simulink model "final_model"  (R2023b)
settings: Solver=VariableStepAuto  StartTime=0.0  StopTime=200  RelTol=1e-3
(part 2 of 3)

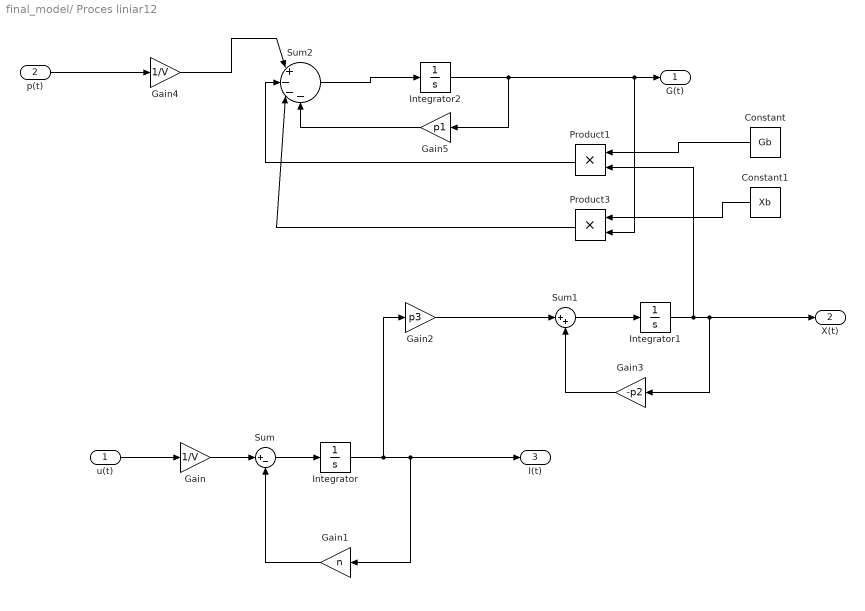
== system final_model/ Proces liniar12 ==
  " u(t)" : Inport
  p(t) : Inport  Port=2
  Constant : Constant  Value=Gb
  Constant1 : Constant  Value=Xb
  Gain : Gain  Gain=1/V
  Gain1 : Gain  Gain=n
  Gain2 : Gain  Gain=p3
  Gain3 : Gain  Gain=-p2
  Gain4 : Gain  Gain=1/V
  Gain5 : Gain  Gain=p1
  Integrator : Integrator
  Integrator1 : Integrator
  Integrator2 : Integrator  InitialCondition=G0
  Product1 : Product
  Product3 : Product
  Sum : Sum  Inputs=|+-
  Sum1 : Sum  Inputs=|++
  Sum2 : Sum  Inputs=|+---
  " G(t)" : Outport
  X(t) : Outport  Port=2
  I(t) : Outport  Port=3
  wires:
  Gain2/1 -> Sum1/1
  Gain/1 -> Sum/1
  " u(t)"/1 -> Gain/1
  Sum/1 -> Integrator/1
  Gain1/1 -> Sum/2
  Integrator2/1 -> Product3/2, " G(t)"/1, Gain5/1
  Integrator1/1 -> Product1/2, Gain3/1, X(t)/1
  Integrator/1 -> Gain2/1, I(t)/1, Gain1/1
  Gain3/1 -> Sum1/2
  Gain4/1 -> Sum2/1
  Gain5/1 -> Sum2/4
  p(t)/1 -> Gain4/1
  Sum1/1 -> Integrator1/1
  Sum2/1 -> Integrator2/1
  Constant/1 -> Product1/1
  Constant1/1 -> Product3/1
  Product3/1 -> Sum2/3
  Product1/1 -> Sum2/2

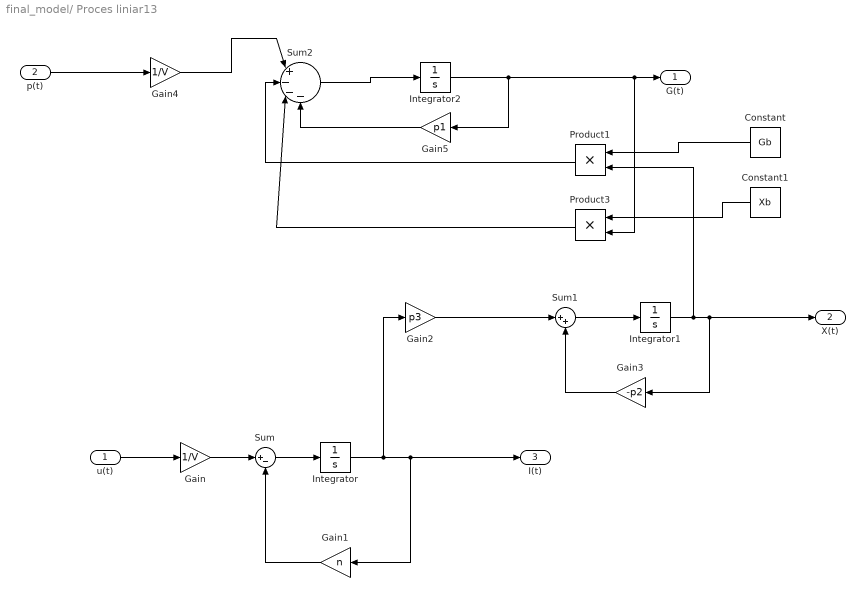
== system final_model/ Proces liniar13 ==
  " u(t)" : Inport
  p(t) : Inport  Port=2
  Constant : Constant  Value=Gb
  Constant1 : Constant  Value=Xb
  Gain : Gain  Gain=1/V
  Gain1 : Gain  Gain=n
  Gain2 : Gain  Gain=p3
  Gain3 : Gain  Gain=-p2
  Gain4 : Gain  Gain=1/V
  Gain5 : Gain  Gain=p1
  Integrator : Integrator
  Integrator1 : Integrator
  Integrator2 : Integrator  InitialCondition=G0
  Product1 : Product
  Product3 : Product
  Sum : Sum  Inputs=|+-
  Sum1 : Sum  Inputs=|++
  Sum2 : Sum  Inputs=|+---
  " G(t)" : Outport
  X(t) : Outport  Port=2
  I(t) : Outport  Port=3
  wires:
  Gain2/1 -> Sum1/1
  Gain/1 -> Sum/1
  " u(t)"/1 -> Gain/1
  Sum/1 -> Integrator/1
  Gain1/1 -> Sum/2
  Integrator2/1 -> Product3/2, " G(t)"/1, Gain5/1
  Integrator1/1 -> Product1/2, Gain3/1, X(t)/1
  Integrator/1 -> Gain2/1, I(t)/1, Gain1/1
  Gain3/1 -> Sum1/2
  Gain4/1 -> Sum2/1
  Gain5/1 -> Sum2/4
  p(t)/1 -> Gain4/1
  Sum1/1 -> Integrator1/1
  Sum2/1 -> Integrator2/1
  Constant/1 -> Product1/1
  Constant1/1 -> Product3/1
  Product3/1 -> Sum2/3
  Product1/1 -> Sum2/2

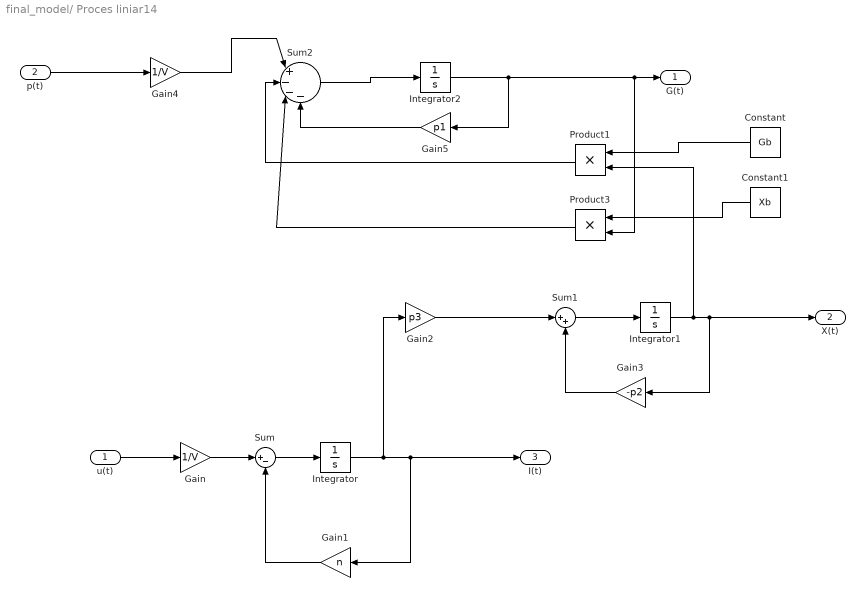
== system final_model/ Proces liniar14 ==
  " u(t)" : Inport
  p(t) : Inport  Port=2
  Constant : Constant  Value=Gb
  Constant1 : Constant  Value=Xb
  Gain : Gain  Gain=1/V
  Gain1 : Gain  Gain=n
  Gain2 : Gain  Gain=p3
  Gain3 : Gain  Gain=-p2
  Gain4 : Gain  Gain=1/V
  Gain5 : Gain  Gain=p1
  Integrator : Integrator
  Integrator1 : Integrator
  Integrator2 : Integrator  InitialCondition=G0
  Product1 : Product
  Product3 : Product
  Sum : Sum  Inputs=|+-
  Sum1 : Sum  Inputs=|++
  Sum2 : Sum  Inputs=|+---
  " G(t)" : Outport
  X(t) : Outport  Port=2
  I(t) : Outport  Port=3
  wires:
  Gain2/1 -> Sum1/1
  Gain/1 -> Sum/1
  " u(t)"/1 -> Gain/1
  Sum/1 -> Integrator/1
  Gain1/1 -> Sum/2
  Integrator2/1 -> Product3/2, " G(t)"/1, Gain5/1
  Integrator1/1 -> Product1/2, Gain3/1, X(t)/1
  Integrator/1 -> Gain2/1, I(t)/1, Gain1/1
  Gain3/1 -> Sum1/2
  Gain4/1 -> Sum2/1
  Gain5/1 -> Sum2/4
  p(t)/1 -> Gain4/1
  Sum1/1 -> Integrator1/1
  Sum2/1 -> Integrator2/1
  Constant/1 -> Product1/1
  Constant1/1 -> Product3/1
  Product3/1 -> Sum2/3
  Product1/1 -> Sum2/2

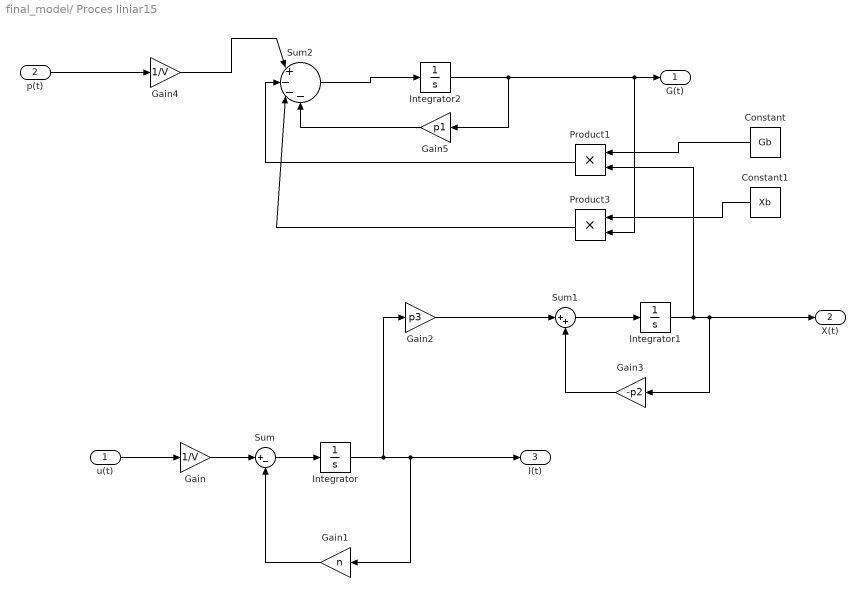
== system final_model/ Proces liniar15 ==
  " u(t)" : Inport
  p(t) : Inport  Port=2
  Constant : Constant  Value=Gb
  Constant1 : Constant  Value=Xb
  Gain : Gain  Gain=1/V
  Gain1 : Gain  Gain=n
  Gain2 : Gain  Gain=p3
  Gain3 : Gain  Gain=-p2
  Gain4 : Gain  Gain=1/V
  Gain5 : Gain  Gain=p1
  Integrator : Integrator
  Integrator1 : Integrator
  Integrator2 : Integrator  InitialCondition=G0
  Product1 : Product
  Product3 : Product
  Sum : Sum  Inputs=|+-
  Sum1 : Sum  Inputs=|++
  Sum2 : Sum  Inputs=|+---
  " G(t)" : Outport
  X(t) : Outport  Port=2
  I(t) : Outport  Port=3
  wires:
  Gain2/1 -> Sum1/1
  Gain/1 -> Sum/1
  " u(t)"/1 -> Gain/1
  Sum/1 -> Integrator/1
  Gain1/1 -> Sum/2
  Integrator2/1 -> Product3/2, " G(t)"/1, Gain5/1
  Integrator1/1 -> Product1/2, Gain3/1, X(t)/1
  Integrator/1 -> Gain2/1, I(t)/1, Gain1/1
  Gain3/1 -> Sum1/2
  Gain4/1 -> Sum2/1
  Gain5/1 -> Sum2/4
  p(t)/1 -> Gain4/1
  Sum1/1 -> Integrator1/1
  Sum2/1 -> Integrator2/1
  Constant/1 -> Product1/1
  Constant1/1 -> Product3/1
  Product3/1 -> Sum2/3
  Product1/1 -> Sum2/2

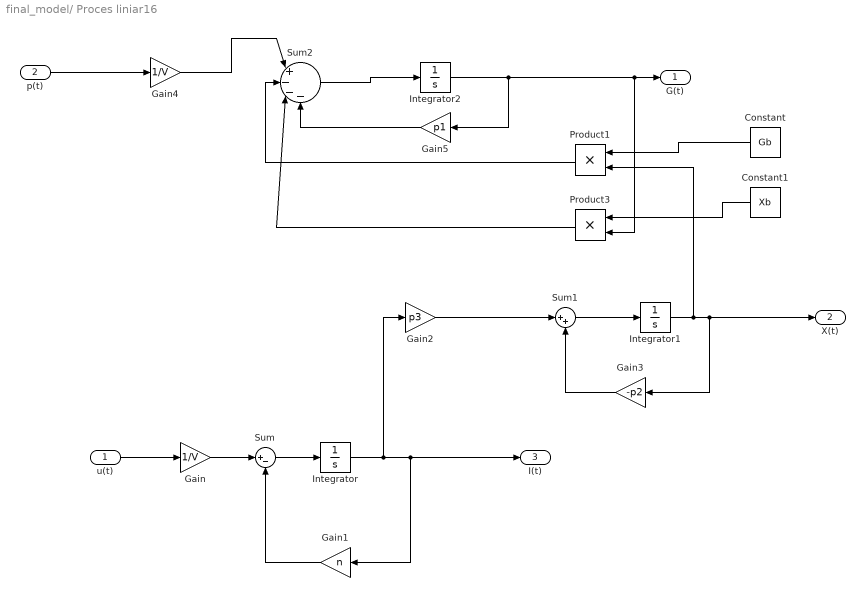
== system final_model/ Proces liniar16 ==
  " u(t)" : Inport
  p(t) : Inport  Port=2
  Constant : Constant  Value=Gb
  Constant1 : Constant  Value=Xb
  Gain : Gain  Gain=1/V
  Gain1 : Gain  Gain=n
  Gain2 : Gain  Gain=p3
  Gain3 : Gain  Gain=-p2
  Gain4 : Gain  Gain=1/V
  Gain5 : Gain  Gain=p1
  Integrator : Integrator
  Integrator1 : Integrator
  Integrator2 : Integrator  InitialCondition=G0
  Product1 : Product
  Product3 : Product
  Sum : Sum  Inputs=|+-
  Sum1 : Sum  Inputs=|++
  Sum2 : Sum  Inputs=|+---
  " G(t)" : Outport
  X(t) : Outport  Port=2
  I(t) : Outport  Port=3
  wires:
  Gain2/1 -> Sum1/1
  Gain/1 -> Sum/1
  " u(t)"/1 -> Gain/1
  Sum/1 -> Integrator/1
  Gain1/1 -> Sum/2
  Integrator2/1 -> Product3/2, " G(t)"/1, Gain5/1
  Integrator1/1 -> Product1/2, Gain3/1, X(t)/1
  Integrator/1 -> Gain2/1, I(t)/1, Gain1/1
  Gain3/1 -> Sum1/2
  Gain4/1 -> Sum2/1
  Gain5/1 -> Sum2/4
  p(t)/1 -> Gain4/1
  Sum1/1 -> Integrator1/1
  Sum2/1 -> Integrator2/1
  Constant/1 -> Product1/1
  Constant1/1 -> Product3/1
  Product3/1 -> Sum2/3
  Product1/1 -> Sum2/2

== system final_model/ Proces liniar17 ==
  " u(t)" : Inport
  p(t) : Inport  Port=2
  Constant : Constant  Value=Gb
  Constant1 : Constant  Value=Xb
  Gain : Gain  Gain=1/V
  Gain1 : Gain  Gain=n
  Gain2 : Gain  Gain=p3
  Gain3 : Gain  Gain=-p2
  Gain4 : Gain  Gain=1/V
  Gain5 : Gain  Gain=p1
  Integrator : Integrator
  Integrator1 : Integrator
  Integrator2 : Integrator  InitialCondition=G0
  Product1 : Product
  Product3 : Product
  Sum : Sum  Inputs=|+-
  Sum1 : Sum  Inputs=|++
  Sum2 : Sum  Inputs=|+---
  " G(t)" : Outport
  X(t) : Outport  Port=2
  I(t) : Outport  Port=3
  wires:
  Gain2/1 -> Sum1/1
  Gain/1 -> Sum/1
  " u(t)"/1 -> Gain/1
  Sum/1 -> Integrator/1
  Gain1/1 -> Sum/2
  Integrator2/1 -> Product3/2, " G(t)"/1, Gain5/1
  Integrator1/1 -> Product1/2, Gain3/1, X(t)/1
  Integrator/1 -> Gain2/1, I(t)/1, Gain1/1
  Gain3/1 -> Sum1/2
  Gain4/1 -> Sum2/1
  Gain5/1 -> Sum2/4
  p(t)/1 -> Gain4/1
  Sum1/1 -> Integrator1/1
  Sum2/1 -> Integrator2/1
  Constant/1 -> Product1/1
  Constant1/1 -> Product3/1
  Product3/1 -> Sum2/3
  Product1/1 -> Sum2/2

== system final_model/ Proces liniar18 ==
  " u(t)" : Inport
  p(t) : Inport  Port=2
  Constant : Constant  Value=Gb
  Constant1 : Constant  Value=Xb
  Gain : Gain  Gain=1/V
  Gain1 : Gain  Gain=n
  Gain2 : Gain  Gain=p3
  Gain3 : Gain  Gain=-p2
  Gain4 : Gain  Gain=1/V
  Gain5 : Gain  Gain=p1
  Integrator : Integrator
  Integrator1 : Integrator
  Integrator2 : Integrator  InitialCondition=G0
  Product1 : Product
  Product3 : Product
  Sum : Sum  Inputs=|+-
  Sum1 : Sum  Inputs=|++
  Sum2 : Sum  Inputs=|+---
  " G(t)" : Outport
  X(t) : Outport  Port=2
  I(t) : Outport  Port=3
  wires:
  Gain2/1 -> Sum1/1
  Gain/1 -> Sum/1
  " u(t)"/1 -> Gain/1
  Sum/1 -> Integrator/1
  Gain1/1 -> Sum/2
  Integrator2/1 -> Product3/2, " G(t)"/1, Gain5/1
  Integrator1/1 -> Product1/2, Gain3/1, X(t)/1
  Integrator/1 -> Gain2/1, I(t)/1, Gain1/1
  Gain3/1 -> Sum1/2
  Gain4/1 -> Sum2/1
  Gain5/1 -> Sum2/4
  p(t)/1 -> Gain4/1
  Sum1/1 -> Integrator1/1
  Sum2/1 -> Integrator2/1
  Constant/1 -> Product1/1
  Constant1/1 -> Product3/1
  Product3/1 -> Sum2/3
  Product1/1 -> Sum2/2

== system final_model/ Proces liniar19 ==
  " u(t)" : Inport
  p(t) : Inport  Port=2
  Constant : Constant  Value=Gb
  Constant1 : Constant  Value=Xb
  Gain : Gain  Gain=1/V
  Gain1 : Gain  Gain=n
  Gain2 : Gain  Gain=p3
  Gain3 : Gain  Gain=-p2
  Gain4 : Gain  Gain=1/V
  Gain5 : Gain  Gain=p1
  Integrator : Integrator
  Integrator1 : Integrator
  Integrator2 : Integrator  InitialCondition=G0
  Product1 : Product
  Product3 : Product
  Sum : Sum  Inputs=|+-
  Sum1 : Sum  Inputs=|++
  Sum2 : Sum  Inputs=|+---
  " G(t)" : Outport
  X(t) : Outport  Port=2
  I(t) : Outport  Port=3
  wires:
  Gain2/1 -> Sum1/1
  Gain/1 -> Sum/1
  " u(t)"/1 -> Gain/1
  Sum/1 -> Integrator/1
  Gain1/1 -> Sum/2
  Integrator2/1 -> Product3/2, " G(t)"/1, Gain5/1
  Integrator1/1 -> Product1/2, Gain3/1, X(t)/1
  Integrator/1 -> Gain2/1, I(t)/1, Gain1/1
  Gain3/1 -> Sum1/2
  Gain4/1 -> Sum2/1
  Gain5/1 -> Sum2/4
  p(t)/1 -> Gain4/1
  Sum1/1 -> Integrator1/1
  Sum2/1 -> Integrator2/1
  Constant/1 -> Product1/1
  Constant1/1 -> Product3/1
  Product3/1 -> Sum2/3
  Product1/1 -> Sum2/2

== system final_model/ Proces liniar2 ==
  " u(t)" : Inport
  p(t) : Inport  Port=2
  Constant : Constant  Value=Gb
  Constant1 : Constant  Value=Xb
  Gain : Gain  Gain=1/V
  Gain1 : Gain  Gain=n
  Gain2 : Gain  Gain=p3
  Gain3 : Gain  Gain=-p2
  Gain4 : Gain  Gain=1/V
  Gain5 : Gain  Gain=p1
  Integrator : Integrator
  Integrator1 : Integrator
  Integrator2 : Integrator  InitialCondition=G0
  Product1 : Product
  Product3 : Product
  Sum : Sum  Inputs=|+-
  Sum1 : Sum  Inputs=|++
  Sum2 : Sum  Inputs=|+---
  " G(t)" : Outport
  X(t) : Outport  Port=2
  I(t) : Outport  Port=3
  wires:
  Gain2/1 -> Sum1/1
  Gain/1 -> Sum/1
  " u(t)"/1 -> Gain/1
  Sum/1 -> Integrator/1
  Gain1/1 -> Sum/2
  Integrator2/1 -> Product3/2, " G(t)"/1, Gain5/1
  Integrator1/1 -> Product1/2, Gain3/1, X(t)/1
  Integrator/1 -> Gain2/1, I(t)/1, Gain1/1
  Gain3/1 -> Sum1/2
  Gain4/1 -> Sum2/1
  Gain5/1 -> Sum2/4
  p(t)/1 -> Gain4/1
  Sum1/1 -> Integrator1/1
  Sum2/1 -> Integrator2/1
  Constant/1 -> Product1/1
  Constant1/1 -> Product3/1
  Product3/1 -> Sum2/3
  Product1/1 -> Sum2/2

== system final_model/ Proces liniar20 ==
  " u(t)" : Inport
  p(t) : Inport  Port=2
  Constant : Constant  Value=Gb
  Constant1 : Constant  Value=Xb
  Gain : Gain  Gain=1/V
  Gain1 : Gain  Gain=n
  Gain2 : Gain  Gain=p3
  Gain3 : Gain  Gain=-p2
  Gain4 : Gain  Gain=1/V
  Gain5 : Gain  Gain=p1
  Integrator : Integrator
  Integrator1 : Integrator
  Integrator2 : Integrator  InitialCondition=G0
  Product1 : Product
  Product3 : Product
  Sum : Sum  Inputs=|+-
  Sum1 : Sum  Inputs=|++
  Sum2 : Sum  Inputs=|+---
  " G(t)" : Outport
  X(t) : Outport  Port=2
  I(t) : Outport  Port=3
  wires:
  Gain2/1 -> Sum1/1
  Gain/1 -> Sum/1
  " u(t)"/1 -> Gain/1
  Sum/1 -> Integrator/1
  Gain1/1 -> Sum/2
  Integrator2/1 -> Product3/2, " G(t)"/1, Gain5/1
  Integrator1/1 -> Product1/2, Gain3/1, X(t)/1
  Integrator/1 -> Gain2/1, I(t)/1, Gain1/1
  Gain3/1 -> Sum1/2
  Gain4/1 -> Sum2/1
  Gain5/1 -> Sum2/4
  p(t)/1 -> Gain4/1
  Sum1/1 -> Integrator1/1
  Sum2/1 -> Integrator2/1
  Constant/1 -> Product1/1
  Constant1/1 -> Product3/1
  Product3/1 -> Sum2/3
  Product1/1 -> Sum2/2

== system final_model/ Proces liniar21 ==
  " u(t)" : Inport
  p(t) : Inport  Port=2
  Constant : Constant  Value=Gb
  Constant1 : Constant  Value=Xb
  Gain : Gain  Gain=1/V
  Gain1 : Gain  Gain=n
  Gain2 : Gain  Gain=p3
  Gain3 : Gain  Gain=-p2
  Gain4 : Gain  Gain=1/V
  Gain5 : Gain  Gain=p1
  Integrator : Integrator
  Integrator1 : Integrator
  Integrator2 : Integrator  InitialCondition=G0
  Product1 : Product
  Product3 : Product
  Sum : Sum  Inputs=|+-
  Sum1 : Sum  Inputs=|++
  Sum2 : Sum  Inputs=|+---
  " G(t)" : Outport
  X(t) : Outport  Port=2
  I(t) : Outport  Port=3
  wires:
  Gain2/1 -> Sum1/1
  Gain/1 -> Sum/1
  " u(t)"/1 -> Gain/1
  Sum/1 -> Integrator/1
  Gain1/1 -> Sum/2
  Integrator2/1 -> Product3/2, " G(t)"/1, Gain5/1
  Integrator1/1 -> Product1/2, Gain3/1, X(t)/1
  Integrator/1 -> Gain2/1, I(t)/1, Gain1/1
  Gain3/1 -> Sum1/2
  Gain4/1 -> Sum2/1
  Gain5/1 -> Sum2/4
  p(t)/1 -> Gain4/1
  Sum1/1 -> Integrator1/1
  Sum2/1 -> Integrator2/1
  Constant/1 -> Product1/1
  Constant1/1 -> Product3/1
  Product3/1 -> Sum2/3
  Product1/1 -> Sum2/2

== system final_model/ Proces liniar22 ==
  " u(t)" : Inport
  p(t) : Inport  Port=2
  Constant : Constant  Value=Gb
  Constant1 : Constant  Value=Xb
  Gain : Gain  Gain=1/V
  Gain1 : Gain  Gain=n
  Gain2 : Gain  Gain=p3
  Gain3 : Gain  Gain=-p2
  Gain4 : Gain  Gain=1/V
  Gain5 : Gain  Gain=p1
  Integrator : Integrator
  Integrator1 : Integrator
  Integrator2 : Integrator  InitialCondition=G0
  Product1 : Product
  Product3 : Product
  Sum : Sum  Inputs=|+-
  Sum1 : Sum  Inputs=|++
  Sum2 : Sum  Inputs=|+---
  " G(t)" : Outport
  X(t) : Outport  Port=2
  I(t) : Outport  Port=3
  wires:
  Gain2/1 -> Sum1/1
  Gain/1 -> Sum/1
  " u(t)"/1 -> Gain/1
  Sum/1 -> Integrator/1
  Gain1/1 -> Sum/2
  Integrator2/1 -> Product3/2, " G(t)"/1, Gain5/1
  Integrator1/1 -> Product1/2, Gain3/1, X(t)/1
  Integrator/1 -> Gain2/1, I(t)/1, Gain1/1
  Gain3/1 -> Sum1/2
  Gain4/1 -> Sum2/1
  Gain5/1 -> Sum2/4
  p(t)/1 -> Gain4/1
  Sum1/1 -> Integrator1/1
  Sum2/1 -> Integrator2/1
  Constant/1 -> Product1/1
  Constant1/1 -> Product3/1
  Product3/1 -> Sum2/3
  Product1/1 -> Sum2/2

== system final_model/ Proces liniar23 ==
  " u(t)" : Inport
  p(t) : Inport  Port=2
  Constant : Constant  Value=Gb
  Constant1 : Constant  Value=Xb
  Gain : Gain  Gain=1/V
  Gain1 : Gain  Gain=n
  Gain2 : Gain  Gain=p3
  Gain3 : Gain  Gain=-p2
  Gain4 : Gain  Gain=1/V
  Gain5 : Gain  Gain=p1
  Integrator : Integrator
  Integrator1 : Integrator
  Integrator2 : Integrator  InitialCondition=G0
  Product1 : Product
  Product3 : Product
  Sum : Sum  Inputs=|+-
  Sum1 : Sum  Inputs=|++
  Sum2 : Sum  Inputs=|+---
  " G(t)" : Outport
  X(t) : Outport  Port=2
  I(t) : Outport  Port=3
  wires:
  Gain2/1 -> Sum1/1
  Gain/1 -> Sum/1
  " u(t)"/1 -> Gain/1
  Sum/1 -> Integrator/1
  Gain1/1 -> Sum/2
  Integrator2/1 -> Product3/2, " G(t)"/1, Gain5/1
  Integrator1/1 -> Product1/2, Gain3/1, X(t)/1
  Integrator/1 -> Gain2/1, I(t)/1, Gain1/1
  Gain3/1 -> Sum1/2
  Gain4/1 -> Sum2/1
  Gain5/1 -> Sum2/4
  p(t)/1 -> Gain4/1
  Sum1/1 -> Integrator1/1
  Sum2/1 -> Integrator2/1
  Constant/1 -> Product1/1
  Constant1/1 -> Product3/1
  Product3/1 -> Sum2/3
  Product1/1 -> Sum2/2

== system final_model/ Proces liniar24 ==
  " u(t)" : Inport
  p(t) : Inport  Port=2
  Constant : Constant  Value=Gb
  Constant1 : Constant  Value=Xb
  Gain : Gain  Gain=1/V
  Gain1 : Gain  Gain=n
  Gain2 : Gain  Gain=p3
  Gain3 : Gain  Gain=-p2
  Gain4 : Gain  Gain=1/V
  Gain5 : Gain  Gain=p1
  Integrator : Integrator
  Integrator1 : Integrator
  Integrator2 : Integrator  InitialCondition=G0
  Product1 : Product
  Product3 : Product
  Sum : Sum  Inputs=|+-
  Sum1 : Sum  Inputs=|++
  Sum2 : Sum  Inputs=|+---
  " G(t)" : Outport
  X(t) : Outport  Port=2
  I(t) : Outport  Port=3
  wires:
  Gain2/1 -> Sum1/1
  Gain/1 -> Sum/1
  " u(t)"/1 -> Gain/1
  Sum/1 -> Integrator/1
  Gain1/1 -> Sum/2
  Integrator2/1 -> Product3/2, " G(t)"/1, Gain5/1
  Integrator1/1 -> Product1/2, Gain3/1, X(t)/1
  Integrator/1 -> Gain2/1, I(t)/1, Gain1/1
  Gain3/1 -> Sum1/2
  Gain4/1 -> Sum2/1
  Gain5/1 -> Sum2/4
  p(t)/1 -> Gain4/1
  Sum1/1 -> Integrator1/1
  Sum2/1 -> Integrator2/1
  Constant/1 -> Product1/1
  Constant1/1 -> Product3/1
  Product3/1 -> Sum2/3
  Product1/1 -> Sum2/2

== system final_model/ Proces liniar25 ==
  " u(t)" : Inport
  p(t) : Inport  Port=2
  Constant : Constant  Value=Gb
  Constant1 : Constant  Value=Xb
  Gain : Gain  Gain=1/V
  Gain1 : Gain  Gain=n
  Gain2 : Gain  Gain=p3
  Gain3 : Gain  Gain=-p2
  Gain4 : Gain  Gain=1/V
  Gain5 : Gain  Gain=p1
  Integrator : Integrator
  Integrator1 : Integrator
  Integrator2 : Integrator  InitialCondition=G0
  Product1 : Product
  Product3 : Product
  Sum : Sum  Inputs=|+-
  Sum1 : Sum  Inputs=|++
  Sum2 : Sum  Inputs=|+---
  " G(t)" : Outport
  X(t) : Outport  Port=2
  I(t) : Outport  Port=3
  wires:
  Gain2/1 -> Sum1/1
  Gain/1 -> Sum/1
  " u(t)"/1 -> Gain/1
  Sum/1 -> Integrator/1
  Gain1/1 -> Sum/2
  Integrator2/1 -> Product3/2, " G(t)"/1, Gain5/1
  Integrator1/1 -> Product1/2, Gain3/1, X(t)/1
  Integrator/1 -> Gain2/1, I(t)/1, Gain1/1
  Gain3/1 -> Sum1/2
  Gain4/1 -> Sum2/1
  Gain5/1 -> Sum2/4
  p(t)/1 -> Gain4/1
  Sum1/1 -> Integrator1/1
  Sum2/1 -> Integrator2/1
  Constant/1 -> Product1/1
  Constant1/1 -> Product3/1
  Product3/1 -> Sum2/3
  Product1/1 -> Sum2/2

== system final_model/ Proces liniar26 ==
  " u(t)" : Inport
  p(t) : Inport  Port=2
  Constant : Constant  Value=Gb
  Constant1 : Constant  Value=Xb
  Gain : Gain  Gain=1/V
  Gain1 : Gain  Gain=n
  Gain2 : Gain  Gain=p3
  Gain3 : Gain  Gain=-p2
  Gain4 : Gain  Gain=1/V
  Gain5 : Gain  Gain=p1
  Integrator : Integrator
  Integrator1 : Integrator
  Integrator2 : Integrator  InitialCondition=G0
  Product1 : Product
  Product3 : Product
  Sum : Sum  Inputs=|+-
  Sum1 : Sum  Inputs=|++
  Sum2 : Sum  Inputs=|+---
  " G(t)" : Outport
  X(t) : Outport  Port=2
  I(t) : Outport  Port=3
  wires:
  Gain2/1 -> Sum1/1
  Gain/1 -> Sum/1
  " u(t)"/1 -> Gain/1
  Sum/1 -> Integrator/1
  Gain1/1 -> Sum/2
  Integrator2/1 -> Product3/2, " G(t)"/1, Gain5/1
  Integrator1/1 -> Product1/2, Gain3/1, X(t)/1
  Integrator/1 -> Gain2/1, I(t)/1, Gain1/1
  Gain3/1 -> Sum1/2
  Gain4/1 -> Sum2/1
  Gain5/1 -> Sum2/4
  p(t)/1 -> Gain4/1
  Sum1/1 -> Integrator1/1
  Sum2/1 -> Integrator2/1
  Constant/1 -> Product1/1
  Constant1/1 -> Product3/1
  Product3/1 -> Sum2/3
  Product1/1 -> Sum2/2

== system final_model/ Proces liniar27 ==
  " u(t)" : Inport
  p(t) : Inport  Port=2
  Constant : Constant  Value=Gb
  Constant1 : Constant  Value=Xb
  Gain : Gain  Gain=1/V
  Gain1 : Gain  Gain=n
  Gain2 : Gain  Gain=p3
  Gain3 : Gain  Gain=-p2
  Gain4 : Gain  Gain=1/V
  Gain5 : Gain  Gain=p1
  Integrator : Integrator
  Integrator1 : Integrator
  Integrator2 : Integrator  InitialCondition=G0
  Product1 : Product
  Product3 : Product
  Sum : Sum  Inputs=|+-
  Sum1 : Sum  Inputs=|++
  Sum2 : Sum  Inputs=|+---
  " G(t)" : Outport
  X(t) : Outport  Port=2
  I(t) : Outport  Port=3
  wires:
  Gain2/1 -> Sum1/1
  Gain/1 -> Sum/1
  " u(t)"/1 -> Gain/1
  Sum/1 -> Integrator/1
  Gain1/1 -> Sum/2
  Integrator2/1 -> Product3/2, " G(t)"/1, Gain5/1
  Integrator1/1 -> Product1/2, Gain3/1, X(t)/1
  Integrator/1 -> Gain2/1, I(t)/1, Gain1/1
  Gain3/1 -> Sum1/2
  Gain4/1 -> Sum2/1
  Gain5/1 -> Sum2/4
  p(t)/1 -> Gain4/1
  Sum1/1 -> Integrator1/1
  Sum2/1 -> Integrator2/1
  Constant/1 -> Product1/1
  Constant1/1 -> Product3/1
  Product3/1 -> Sum2/3
  Product1/1 -> Sum2/2

== system final_model/ Proces liniar28 ==
  " u(t)" : Inport
  p(t) : Inport  Port=2
  Constant : Constant  Value=Gb
  Constant1 : Constant  Value=Xb
  Gain : Gain  Gain=1/V
  Gain1 : Gain  Gain=n
  Gain2 : Gain  Gain=p3
  Gain3 : Gain  Gain=-p2
  Gain4 : Gain  Gain=1/V
  Gain5 : Gain  Gain=p1
  Integrator : Integrator
  Integrator1 : Integrator
  Integrator2 : Integrator  InitialCondition=G0
  Product1 : Product
  Product3 : Product
  Sum : Sum  Inputs=|+-
  Sum1 : Sum  Inputs=|++
  Sum2 : Sum  Inputs=|+---
  " G(t)" : Outport
  X(t) : Outport  Port=2
  I(t) : Outport  Port=3
  wires:
  Gain2/1 -> Sum1/1
  Gain/1 -> Sum/1
  " u(t)"/1 -> Gain/1
  Sum/1 -> Integrator/1
  Gain1/1 -> Sum/2
  Integrator2/1 -> Product3/2, " G(t)"/1, Gain5/1
  Integrator1/1 -> Product1/2, Gain3/1, X(t)/1
  Integrator/1 -> Gain2/1, I(t)/1, Gain1/1
  Gain3/1 -> Sum1/2
  Gain4/1 -> Sum2/1
  Gain5/1 -> Sum2/4
  p(t)/1 -> Gain4/1
  Sum1/1 -> Integrator1/1
  Sum2/1 -> Integrator2/1
  Constant/1 -> Product1/1
  Constant1/1 -> Product3/1
  Product3/1 -> Sum2/3
  Product1/1 -> Sum2/2

== system final_model/ Proces liniar29 ==
  " u(t)" : Inport
  p(t) : Inport  Port=2
  Constant : Constant  Value=Gb
  Constant1 : Constant  Value=Xb
  Gain : Gain  Gain=1/V
  Gain1 : Gain  Gain=n
  Gain2 : Gain  Gain=p3
  Gain3 : Gain  Gain=-p2
  Gain4 : Gain  Gain=1/V
  Gain5 : Gain  Gain=p1
  Integrator : Integrator
  Integrator1 : Integrator
  Integrator2 : Integrator  InitialCondition=G0
  Product1 : Product
  Product3 : Product
  Sum : Sum  Inputs=|+-
  Sum1 : Sum  Inputs=|++
  Sum2 : Sum  Inputs=|+---
  " G(t)" : Outport
  X(t) : Outport  Port=2
  I(t) : Outport  Port=3
  wires:
  Gain2/1 -> Sum1/1
  Gain/1 -> Sum/1
  " u(t)"/1 -> Gain/1
  Sum/1 -> Integrator/1
  Gain1/1 -> Sum/2
  Integrator2/1 -> Product3/2, " G(t)"/1, Gain5/1
  Integrator1/1 -> Product1/2, Gain3/1, X(t)/1
  Integrator/1 -> Gain2/1, I(t)/1, Gain1/1
  Gain3/1 -> Sum1/2
  Gain4/1 -> Sum2/1
  Gain5/1 -> Sum2/4
  p(t)/1 -> Gain4/1
  Sum1/1 -> Integrator1/1
  Sum2/1 -> Integrator2/1
  Constant/1 -> Product1/1
  Constant1/1 -> Product3/1
  Product3/1 -> Sum2/3
  Product1/1 -> Sum2/2

== system final_model/ Proces liniar3 ==
  " u(t)" : Inport
  p(t) : Inport  Port=2
  Constant : Constant  Value=Gb
  Constant1 : Constant  Value=Xb
  Gain : Gain  Gain=1/V
  Gain1 : Gain  Gain=n
  Gain2 : Gain  Gain=p3
  Gain3 : Gain  Gain=-p2
  Gain4 : Gain  Gain=1/V
  Gain5 : Gain  Gain=p1
  Integrator : Integrator
  Integrator1 : Integrator
  Integrator2 : Integrator  InitialCondition=G0
  Product1 : Product
  Product3 : Product
  Sum : Sum  Inputs=|+-
  Sum1 : Sum  Inputs=|++
  Sum2 : Sum  Inputs=|+---
  " G(t)" : Outport
  X(t) : Outport  Port=2
  I(t) : Outport  Port=3
  wires:
  Gain2/1 -> Sum1/1
  Gain/1 -> Sum/1
  " u(t)"/1 -> Gain/1
  Sum/1 -> Integrator/1
  Gain1/1 -> Sum/2
  Integrator2/1 -> Product3/2, " G(t)"/1, Gain5/1
  Integrator1/1 -> Product1/2, Gain3/1, X(t)/1
  Integrator/1 -> Gain2/1, I(t)/1, Gain1/1
  Gain3/1 -> Sum1/2
  Gain4/1 -> Sum2/1
  Gain5/1 -> Sum2/4
  p(t)/1 -> Gain4/1
  Sum1/1 -> Integrator1/1
  Sum2/1 -> Integrator2/1
  Constant/1 -> Product1/1
  Constant1/1 -> Product3/1
  Product3/1 -> Sum2/3
  Product1/1 -> Sum2/2

== system final_model/ Proces liniar30 ==
  " u(t)" : Inport
  p(t) : Inport  Port=2
  Constant : Constant  Value=Gb
  Constant1 : Constant  Value=Xb
  Gain : Gain  Gain=1/V
  Gain1 : Gain  Gain=n
  Gain2 : Gain  Gain=p3
  Gain3 : Gain  Gain=-p2
  Gain4 : Gain  Gain=1/V
  Gain5 : Gain  Gain=p1
  Integrator : Integrator
  Integrator1 : Integrator
  Integrator2 : Integrator  InitialCondition=G0
  Product1 : Product
  Product3 : Product
  Sum : Sum  Inputs=|+-
  Sum1 : Sum  Inputs=|++
  Sum2 : Sum  Inputs=|+---
  " G(t)" : Outport
  X(t) : Outport  Port=2
  I(t) : Outport  Port=3
  wires:
  Gain2/1 -> Sum1/1
  Gain/1 -> Sum/1
  " u(t)"/1 -> Gain/1
  Sum/1 -> Integrator/1
  Gain1/1 -> Sum/2
  Integrator2/1 -> Product3/2, " G(t)"/1, Gain5/1
  Integrator1/1 -> Product1/2, Gain3/1, X(t)/1
  Integrator/1 -> Gain2/1, I(t)/1, Gain1/1
  Gain3/1 -> Sum1/2
  Gain4/1 -> Sum2/1
  Gain5/1 -> Sum2/4
  p(t)/1 -> Gain4/1
  Sum1/1 -> Integrator1/1
  Sum2/1 -> Integrator2/1
  Constant/1 -> Product1/1
  Constant1/1 -> Product3/1
  Product3/1 -> Sum2/3
  Product1/1 -> Sum2/2

== system final_model/ Proces liniar4 ==
  " u(t)" : Inport
  p(t) : Inport  Port=2
  Constant : Constant  Value=Gb
  Constant1 : Constant  Value=Xb
  Gain : Gain  Gain=1/V
  Gain1 : Gain  Gain=n
  Gain2 : Gain  Gain=p3
  Gain3 : Gain  Gain=-p2
  Gain4 : Gain  Gain=1/V
  Gain5 : Gain  Gain=p1
  Integrator : Integrator
  Integrator1 : Integrator
  Integrator2 : Integrator  InitialCondition=G0
  Product1 : Product
  Product3 : Product
  Sum : Sum  Inputs=|+-
  Sum1 : Sum  Inputs=|++
  Sum2 : Sum  Inputs=|+---
  " G(t)" : Outport
  X(t) : Outport  Port=2
  I(t) : Outport  Port=3
  wires:
  Gain2/1 -> Sum1/1
  Gain/1 -> Sum/1
  " u(t)"/1 -> Gain/1
  Sum/1 -> Integrator/1
  Gain1/1 -> Sum/2
  Integrator2/1 -> Product3/2, " G(t)"/1, Gain5/1
  Integrator1/1 -> Product1/2, Gain3/1, X(t)/1
  Integrator/1 -> Gain2/1, I(t)/1, Gain1/1
  Gain3/1 -> Sum1/2
  Gain4/1 -> Sum2/1
  Gain5/1 -> Sum2/4
  p(t)/1 -> Gain4/1
  Sum1/1 -> Integrator1/1
  Sum2/1 -> Integrator2/1
  Constant/1 -> Product1/1
  Constant1/1 -> Product3/1
  Product3/1 -> Sum2/3
  Product1/1 -> Sum2/2

== system final_model/ Proces liniar5 ==
  " u(t)" : Inport
  p(t) : Inport  Port=2
  Constant : Constant  Value=Gb
  Constant1 : Constant  Value=Xb
  Gain : Gain  Gain=1/V
  Gain1 : Gain  Gain=n
  Gain2 : Gain  Gain=p3
  Gain3 : Gain  Gain=-p2
  Gain4 : Gain  Gain=1/V
  Gain5 : Gain  Gain=p1
  Integrator : Integrator
  Integrator1 : Integrator
  Integrator2 : Integrator  InitialCondition=G0
  Product1 : Product
  Product3 : Product
  Sum : Sum  Inputs=|+-
  Sum1 : Sum  Inputs=|++
  Sum2 : Sum  Inputs=|+---
  " G(t)" : Outport
  X(t) : Outport  Port=2
  I(t) : Outport  Port=3
  wires:
  Gain2/1 -> Sum1/1
  Gain/1 -> Sum/1
  " u(t)"/1 -> Gain/1
  Sum/1 -> Integrator/1
  Gain1/1 -> Sum/2
  Integrator2/1 -> Product3/2, " G(t)"/1, Gain5/1
  Integrator1/1 -> Product1/2, Gain3/1, X(t)/1
  Integrator/1 -> Gain2/1, I(t)/1, Gain1/1
  Gain3/1 -> Sum1/2
  Gain4/1 -> Sum2/1
  Gain5/1 -> Sum2/4
  p(t)/1 -> Gain4/1
  Sum1/1 -> Integrator1/1
  Sum2/1 -> Integrator2/1
  Constant/1 -> Product1/1
  Constant1/1 -> Product3/1
  Product3/1 -> Sum2/3
  Product1/1 -> Sum2/2

== system final_model/ Proces liniar6 ==
  " u(t)" : Inport
  p(t) : Inport  Port=2
  Constant : Constant  Value=Gb
  Constant1 : Constant  Value=Xb
  Gain : Gain  Gain=1/V
  Gain1 : Gain  Gain=n
  Gain2 : Gain  Gain=p3
  Gain3 : Gain  Gain=-p2
  Gain4 : Gain  Gain=1/V
  Gain5 : Gain  Gain=p1
  Integrator : Integrator
  Integrator1 : Integrator
  Integrator2 : Integrator  InitialCondition=G0
  Product1 : Product
  Product3 : Product
  Sum : Sum  Inputs=|+-
  Sum1 : Sum  Inputs=|++
  Sum2 : Sum  Inputs=|+---
  " G(t)" : Outport
  X(t) : Outport  Port=2
  I(t) : Outport  Port=3
  wires:
  Gain2/1 -> Sum1/1
  Gain/1 -> Sum/1
  " u(t)"/1 -> Gain/1
  Sum/1 -> Integrator/1
  Gain1/1 -> Sum/2
  Integrator2/1 -> Product3/2, " G(t)"/1, Gain5/1
  Integrator1/1 -> Product1/2, Gain3/1, X(t)/1
  Integrator/1 -> Gain2/1, I(t)/1, Gain1/1
  Gain3/1 -> Sum1/2
  Gain4/1 -> Sum2/1
  Gain5/1 -> Sum2/4
  p(t)/1 -> Gain4/1
  Sum1/1 -> Integrator1/1
  Sum2/1 -> Integrator2/1
  Constant/1 -> Product1/1
  Constant1/1 -> Product3/1
  Product3/1 -> Sum2/3
  Product1/1 -> Sum2/2

== system final_model/ Proces liniar7 ==
  " u(t)" : Inport
  p(t) : Inport  Port=2
  Constant : Constant  Value=Gb
  Constant1 : Constant  Value=Xb
  Gain : Gain  Gain=1/V
  Gain1 : Gain  Gain=n
  Gain2 : Gain  Gain=p3
  Gain3 : Gain  Gain=-p2
  Gain4 : Gain  Gain=1/V
  Gain5 : Gain  Gain=p1
  Integrator : Integrator
  Integrator1 : Integrator
  Integrator2 : Integrator  InitialCondition=G0
  Product1 : Product
  Product3 : Product
  Sum : Sum  Inputs=|+-
  Sum1 : Sum  Inputs=|++
  Sum2 : Sum  Inputs=|+---
  " G(t)" : Outport
  X(t) : Outport  Port=2
  I(t) : Outport  Port=3
  wires:
  Gain2/1 -> Sum1/1
  Gain/1 -> Sum/1
  " u(t)"/1 -> Gain/1
  Sum/1 -> Integrator/1
  Gain1/1 -> Sum/2
  Integrator2/1 -> Product3/2, " G(t)"/1, Gain5/1
  Integrator1/1 -> Product1/2, Gain3/1, X(t)/1
  Integrator/1 -> Gain2/1, I(t)/1, Gain1/1
  Gain3/1 -> Sum1/2
  Gain4/1 -> Sum2/1
  Gain5/1 -> Sum2/4
  p(t)/1 -> Gain4/1
  Sum1/1 -> Integrator1/1
  Sum2/1 -> Integrator2/1
  Constant/1 -> Product1/1
  Constant1/1 -> Product3/1
  Product3/1 -> Sum2/3
  Product1/1 -> Sum2/2

== system final_model/ Proces liniar8 ==
  " u(t)" : Inport
  p(t) : Inport  Port=2
  Constant : Constant  Value=Gb
  Constant1 : Constant  Value=Xb
  Gain : Gain  Gain=1/V
  Gain1 : Gain  Gain=n
  Gain2 : Gain  Gain=p3
  Gain3 : Gain  Gain=-p2
  Gain4 : Gain  Gain=1/V
  Gain5 : Gain  Gain=p1
  Integrator : Integrator
  Integrator1 : Integrator
  Integrator2 : Integrator  InitialCondition=G0
  Product1 : Product
  Product3 : Product
  Sum : Sum  Inputs=|+-
  Sum1 : Sum  Inputs=|++
  Sum2 : Sum  Inputs=|+---
  " G(t)" : Outport
  X(t) : Outport  Port=2
  I(t) : Outport  Port=3
  wires:
  Gain2/1 -> Sum1/1
  Gain/1 -> Sum/1
  " u(t)"/1 -> Gain/1
  Sum/1 -> Integrator/1
  Gain1/1 -> Sum/2
  Integrator2/1 -> Product3/2, " G(t)"/1, Gain5/1
  Integrator1/1 -> Product1/2, Gain3/1, X(t)/1
  Integrator/1 -> Gain2/1, I(t)/1, Gain1/1
  Gain3/1 -> Sum1/2
  Gain4/1 -> Sum2/1
  Gain5/1 -> Sum2/4
  p(t)/1 -> Gain4/1
  Sum1/1 -> Integrator1/1
  Sum2/1 -> Integrator2/1
  Constant/1 -> Product1/1
  Constant1/1 -> Product3/1
  Product3/1 -> Sum2/3
  Product1/1 -> Sum2/2

== system final_model/ Proces liniar9 ==
  " u(t)" : Inport
  p(t) : Inport  Port=2
  Constant : Constant  Value=Gb
  Constant1 : Constant  Value=Xb
  Gain : Gain  Gain=1/V
  Gain1 : Gain  Gain=n
  Gain2 : Gain  Gain=p3
  Gain3 : Gain  Gain=-p2
  Gain4 : Gain  Gain=1/V
  Gain5 : Gain  Gain=p1
  Integrator : Integrator
  Integrator1 : Integrator
  Integrator2 : Integrator  InitialCondition=G0
  Product1 : Product
  Product3 : Product
  Sum : Sum  Inputs=|+-
  Sum1 : Sum  Inputs=|++
  Sum2 : Sum  Inputs=|+---
  " G(t)" : Outport
  X(t) : Outport  Port=2
  I(t) : Outport  Port=3
  wires:
  Gain2/1 -> Sum1/1
  Gain/1 -> Sum/1
  " u(t)"/1 -> Gain/1
  Sum/1 -> Integrator/1
  Gain1/1 -> Sum/2
  Integrator2/1 -> Product3/2, " G(t)"/1, Gain5/1
  Integrator1/1 -> Product1/2, Gain3/1, X(t)/1
  Integrator/1 -> Gain2/1, I(t)/1, Gain1/1
  Gain3/1 -> Sum1/2
  Gain4/1 -> Sum2/1
  Gain5/1 -> Sum2/4
  p(t)/1 -> Gain4/1
  Sum1/1 -> Integrator1/1
  Sum2/1 -> Integrator2/1
  Constant/1 -> Product1/1
  Constant1/1 -> Product3/1
  Product3/1 -> Sum2/3
  Product1/1 -> Sum2/2

== system final_model/ Proces neliniar ==
  " u(t)" : Inport
  p(t) : Inport  Port=2
  Constant : Constant  Value=p1*Gb
  Constant1 : Constant  Value=p1
  Gain : Gain  Gain=1/V
  Gain1 : Gain  Gain=n
  Gain2 : Gain  Gain=p3
  Gain3 : Gain  Gain=-p2
  Gain4 : Gain  Gain=1/V
  Integrator : Integrator
  Integrator1 : Integrator
  Integrator2 : Integrator  InitialCondition=G0
  Product : Product
  Sum : Sum  Inputs=|+-
  Sum1 : Sum  Inputs=|++
  Sum2 : Sum  Inputs=|++-
  Sum3 : Sum  Inputs=|++
  " G(t)" : Outport
  X(t) : Outport  Port=2
  I(t) : Outport  Port=3
  wires:
  " u(t)"/1 -> Gain/1
  Gain/1 -> Sum/1
  Sum/1 -> Integrator/1
  Integrator/1 -> Gain2/1, I(t)/1, Gain1/1
  Gain1/1 -> Sum/2
  Gain2/1 -> Sum1/1
  Gain3/1 -> Sum1/2
  Integrator1/1 -> Gain3/1, Sum3/2, X(t)/1
  p(t)/1 -> Gain4/1
  Gain4/1 -> Sum2/1
  Constant/1 -> Sum2/2
  Constant1/1 -> Sum3/1
  Sum2/1 -> Integrator2/1
  Product/1 -> Sum2/3
  Sum3/1 -> Product/2
  Integrator2/1 -> Product/1, " G(t)"/1
  Sum1/1 -> Integrator1/1

== system final_model/ Proces neliniar1 ==
  " u(t)" : Inport
  p(t) : Inport  Port=2
  Constant : Constant  Value=p1*Gb
  Constant1 : Constant  Value=p1
  Gain : Gain  Gain=1/V
  Gain1 : Gain  Gain=n
  Gain2 : Gain  Gain=p3
  Gain3 : Gain  Gain=-p2
  Gain4 : Gain  Gain=1/V
  Integrator : Integrator
  Integrator1 : Integrator
  Integrator2 : Integrator  InitialCondition=G0
  Product : Product
  Sum : Sum  Inputs=|+-
  Sum1 : Sum  Inputs=|++
  Sum2 : Sum  Inputs=|++-
  Sum3 : Sum  Inputs=|++
  " G(t)" : Outport
  X(t) : Outport  Port=2
  I(t) : Outport  Port=3
  wires:
  " u(t)"/1 -> Gain/1
  Gain/1 -> Sum/1
  Sum/1 -> Integrator/1
  Integrator/1 -> Gain2/1, I(t)/1, Gain1/1
  Gain1/1 -> Sum/2
  Gain2/1 -> Sum1/1
  Gain3/1 -> Sum1/2
  Integrator1/1 -> Gain3/1, Sum3/2, X(t)/1
  p(t)/1 -> Gain4/1
  Gain4/1 -> Sum2/1
  Constant/1 -> Sum2/2
  Constant1/1 -> Sum3/1
  Sum2/1 -> Integrator2/1
  Product/1 -> Sum2/3
  Sum3/1 -> Product/2
  Integrator2/1 -> Product/1, " G(t)"/1
  Sum1/1 -> Integrator1/1

== system final_model/ Proces neliniar2 ==
  " u(t)" : Inport
  p(t) : Inport  Port=2
  Constant : Constant  Value=p1*Gb
  Constant1 : Constant  Value=p1
  Gain : Gain  Gain=1/V
  Gain1 : Gain  Gain=n
  Gain2 : Gain  Gain=p3
  Gain3 : Gain  Gain=-p2
  Gain4 : Gain  Gain=1/V
  Integrator : Integrator
  Integrator1 : Integrator
  Integrator2 : Integrator  InitialCondition=G0
  Product : Product
  Sum : Sum  Inputs=|+-
  Sum1 : Sum  Inputs=|++
  Sum2 : Sum  Inputs=|++-
  Sum3 : Sum  Inputs=|++
  " G(t)" : Outport
  X(t) : Outport  Port=2
  I(t) : Outport  Port=3
  wires:
  " u(t)"/1 -> Gain/1
  Gain/1 -> Sum/1
  Sum/1 -> Integrator/1
  Integrator/1 -> Gain2/1, I(t)/1, Gain1/1
  Gain1/1 -> Sum/2
  Gain2/1 -> Sum1/1
  Gain3/1 -> Sum1/2
  Integrator1/1 -> Gain3/1, Sum3/2, X(t)/1
  p(t)/1 -> Gain4/1
  Gain4/1 -> Sum2/1
  Constant/1 -> Sum2/2
  Constant1/1 -> Sum3/1
  Sum2/1 -> Integrator2/1
  Product/1 -> Sum2/3
  Sum3/1 -> Product/2
  Integrator2/1 -> Product/1, " G(t)"/1
  Sum1/1 -> Integrator1/1

== system final_model/ Proces neliniar3 ==
  " u(t)" : Inport
  p(t) : Inport  Port=2
  Constant : Constant  Value=p1*Gb
  Constant1 : Constant  Value=p1
  Gain : Gain  Gain=1/V
  Gain1 : Gain  Gain=n
  Gain2 : Gain  Gain=p3
  Gain3 : Gain  Gain=-p2
  Gain4 : Gain  Gain=1/V
  Integrator : Integrator
  Integrator1 : Integrator
  Integrator2 : Integrator  InitialCondition=G0
  Product : Product
  Sum : Sum  Inputs=|+-
  Sum1 : Sum  Inputs=|++
  Sum2 : Sum  Inputs=|++-
  Sum3 : Sum  Inputs=|++
  " G(t)" : Outport
  X(t) : Outport  Port=2
  I(t) : Outport  Port=3
  wires:
  " u(t)"/1 -> Gain/1
  Gain/1 -> Sum/1
  Sum/1 -> Integrator/1
  Integrator/1 -> Gain2/1, I(t)/1, Gain1/1
  Gain1/1 -> Sum/2
  Gain2/1 -> Sum1/1
  Gain3/1 -> Sum1/2
  Integrator1/1 -> Gain3/1, Sum3/2, X(t)/1
  p(t)/1 -> Gain4/1
  Gain4/1 -> Sum2/1
  Constant/1 -> Sum2/2
  Constant1/1 -> Sum3/1
  Sum2/1 -> Integrator2/1
  Product/1 -> Sum2/3
  Sum3/1 -> Product/2
  Integrator2/1 -> Product/1, " G(t)"/1
  Sum1/1 -> Integrator1/1

== system final_model/ Proces neliniar4 ==
  " u(t)" : Inport
  p(t) : Inport  Port=2
  Constant : Constant  Value=p1*Gb
  Constant1 : Constant  Value=p1
  Gain : Gain  Gain=1/V
  Gain1 : Gain  Gain=n
  Gain2 : Gain  Gain=p3
  Gain3 : Gain  Gain=-p2
  Gain4 : Gain  Gain=1/V
  Integrator : Integrator
  Integrator1 : Integrator
  Integrator2 : Integrator  InitialCondition=G0
  Product : Product
  Sum : Sum  Inputs=|+-
  Sum1 : Sum  Inputs=|++
  Sum2 : Sum  Inputs=|++-
  Sum3 : Sum  Inputs=|++
  " G(t)" : Outport
  X(t) : Outport  Port=2
  I(t) : Outport  Port=3
  wires:
  " u(t)"/1 -> Gain/1
  Gain/1 -> Sum/1
  Sum/1 -> Integrator/1
  Integrator/1 -> Gain2/1, I(t)/1, Gain1/1
  Gain1/1 -> Sum/2
  Gain2/1 -> Sum1/1
  Gain3/1 -> Sum1/2
  Integrator1/1 -> Gain3/1, Sum3/2, X(t)/1
  p(t)/1 -> Gain4/1
  Gain4/1 -> Sum2/1
  Constant/1 -> Sum2/2
  Constant1/1 -> Sum3/1
  Sum2/1 -> Integrator2/1
  Product/1 -> Sum2/3
  Sum3/1 -> Product/2
  Integrator2/1 -> Product/1, " G(t)"/1
  Sum1/1 -> Integrator1/1

== system final_model/ Proces neliniar5 ==
  " u(t)" : Inport
  p(t) : Inport  Port=2
  Constant : Constant  Value=p1*Gb
  Constant1 : Constant  Value=p1
  Gain : Gain  Gain=1/V
  Gain1 : Gain  Gain=n
  Gain2 : Gain  Gain=p3
  Gain3 : Gain  Gain=-p2
  Gain4 : Gain  Gain=1/V
  Integrator : Integrator
  Integrator1 : Integrator
  Integrator2 : Integrator  InitialCondition=G0
  Product : Product
  Sum : Sum  Inputs=|+-
  Sum1 : Sum  Inputs=|++
  Sum2 : Sum  Inputs=|++-
  Sum3 : Sum  Inputs=|++
  " G(t)" : Outport
  X(t) : Outport  Port=2
  I(t) : Outport  Port=3
  wires:
  " u(t)"/1 -> Gain/1
  Gain/1 -> Sum/1
  Sum/1 -> Integrator/1
  Integrator/1 -> Gain2/1, I(t)/1, Gain1/1
  Gain1/1 -> Sum/2
  Gain2/1 -> Sum1/1
  Gain3/1 -> Sum1/2
  Integrator1/1 -> Gain3/1, Sum3/2, X(t)/1
  p(t)/1 -> Gain4/1
  Gain4/1 -> Sum2/1
  Constant/1 -> Sum2/2
  Constant1/1 -> Sum3/1
  Sum2/1 -> Integrator2/1
  Product/1 -> Sum2/3
  Sum3/1 -> Product/2
  Integrator2/1 -> Product/1, " G(t)"/1
  Sum1/1 -> Integrator1/1

== system final_model/10.1g ==
  p(t) : Inport
  u(t) : Inport  Port=2
  Constant : Constant  Value=Gb
  Constant1 : Constant  Value=p1
  Gain : Gain  Gain=1/V
  Gain1 : Gain  Gain=p1
  Gain2 : Gain  Gain=p2
  Gain3 : Gain  Gain=1/V
  Gain4 : Gain  Gain=n
  Gain5 : Gain  Gain=p3
  Integrator : Integrator  InitialCondition=G0
  Integrator1 : Integrator
  Integrator2 : Integrator
  Product : Product
  Product1 : Product
  Sum : Sum  Inputs=|++--
  Sum1 : Sum  Inputs=|+-
  Sum2 : Sum  Inputs=|+-
  G(t) : Outport
  X(t) : Outport  Port=2
  I(t) : Outport  Port=3
  wires:
  Sum2/1 -> Integrator2/1
  Gain3/1 -> Sum2/1
  Sum1/1 -> Integrator1/1
  Integrator2/1 -> Gain4/1, I(t)/1, Gain5/1
  u(t)/1 -> Gain3/1
  Integrator1/1 -> Product1/2, X(t)/1, Gain2/1
  Product/1 -> Sum/2
  Integrator/1 -> G(t)/1, Gain1/1, Product1/1
  Gain5/1 -> Sum1/1
  Sum/1 -> Integrator/1
  Constant1/1 -> Product/2
  Constant/1 -> Product/1
  Gain4/1 -> Sum2/2
  Gain2/1 -> Sum1/2
  Product1/1 -> Sum/3
  Gain1/1 -> Sum/4
  p(t)/1 -> Gain/1
  Gain/1 -> Sum/1

== system final_model/10.1g1 ==
  p(t) : Inport
  u(t) : Inport  Port=2
  Constant : Constant  Value=Gb
  Constant1 : Constant  Value=p1
  Gain : Gain  Gain=1/V
  Gain1 : Gain  Gain=p1
  Gain2 : Gain  Gain=p2
  Gain3 : Gain  Gain=1/V
  Gain4 : Gain  Gain=n
  Gain5 : Gain  Gain=p3
  Integrator : Integrator  InitialCondition=G0
  Integrator1 : Integrator
  Integrator2 : Integrator
  Product : Product
  Product1 : Product
  Sum : Sum  Inputs=|++--
  Sum1 : Sum  Inputs=|+-
  Sum2 : Sum  Inputs=|+-
  G(t) : Outport
  X(t) : Outport  Port=2
  I(t) : Outport  Port=3
  wires:
  Sum2/1 -> Integrator2/1
  Gain3/1 -> Sum2/1
  Sum1/1 -> Integrator1/1
  Integrator2/1 -> Gain4/1, I(t)/1, Gain5/1
  u(t)/1 -> Gain3/1
  Integrator1/1 -> Product1/2, X(t)/1, Gain2/1
  Product/1 -> Sum/2
  Integrator/1 -> G(t)/1, Gain1/1, Product1/1
  Gain5/1 -> Sum1/1
  Sum/1 -> Integrator/1
  Constant1/1 -> Product/2
  Constant/1 -> Product/1
  Gain4/1 -> Sum2/2
  Gain2/1 -> Sum1/2
  Product1/1 -> Sum/3
  Gain1/1 -> Sum/4
  p(t)/1 -> Gain/1
  Gain/1 -> Sum/1

== system final_model/1001g ==
  " u(t)" : Inport
  p(t) : Inport  Port=2
  Constant : Constant  Value=p1*Gb
  Constant1 : Constant  Value=p1
  Gain : Gain  Gain=1/V
  Gain1 : Gain  Gain=n
  Gain2 : Gain  Gain=p3
  Gain3 : Gain  Gain=-p2
  Gain4 : Gain  Gain=1/V
  Integrator : Integrator
  Integrator1 : Integrator
  Integrator2 : Integrator  InitialCondition=G0
  Product : Product
  Sum : Sum  Inputs=|+-
  Sum1 : Sum  Inputs=|++
  Sum2 : Sum  Inputs=|++-
  Sum3 : Sum  Inputs=|++
  " G(t)" : Outport
  X(t) : Outport  Port=2
  I(t) : Outport  Port=3
  wires:
  " u(t)"/1 -> Gain/1
  Gain/1 -> Sum/1
  Sum/1 -> Integrator/1
  Integrator/1 -> Gain2/1, I(t)/1, Gain1/1
  Gain1/1 -> Sum/2
  Gain2/1 -> Sum1/1
  Gain3/1 -> Sum1/2
  Integrator1/1 -> Gain3/1, Sum3/2, X(t)/1
  p(t)/1 -> Gain4/1
  Gain4/1 -> Sum2/1
  Constant/1 -> Sum2/2
  Constant1/1 -> Sum3/1
  Sum2/1 -> Integrator2/1
  Product/1 -> Sum2/3
  Sum3/1 -> Product/2
  Integrator2/1 -> Product/1, " G(t)"/1
  Sum1/1 -> Integrator1/1

== system final_model/100g ==
  " u(t)" : Inport
  p(t) : Inport  Port=2
  Constant : Constant  Value=p1*Gb
  Constant1 : Constant  Value=p1
  Gain : Gain  Gain=1/V
  Gain1 : Gain  Gain=n
  Gain2 : Gain  Gain=p3
  Gain3 : Gain  Gain=-p2
  Gain4 : Gain  Gain=1/V
  Integrator : Integrator
  Integrator1 : Integrator
  Integrator2 : Integrator  InitialCondition=G0
  Product : Product
  Sum : Sum  Inputs=|+-
  Sum1 : Sum  Inputs=|++
  Sum2 : Sum  Inputs=|++-
  Sum3 : Sum  Inputs=|++
  " G(t)" : Outport
  X(t) : Outport  Port=2
  I(t) : Outport  Port=3
  wires:
  " u(t)"/1 -> Gain/1
  Gain/1 -> Sum/1
  Sum/1 -> Integrator/1
  Integrator/1 -> Gain2/1, I(t)/1, Gain1/1
  Gain1/1 -> Sum/2
  Gain2/1 -> Sum1/1
  Gain3/1 -> Sum1/2
  Integrator1/1 -> Gain3/1, Sum3/2, X(t)/1
  p(t)/1 -> Gain4/1
  Gain4/1 -> Sum2/1
  Constant/1 -> Sum2/2
  Constant1/1 -> Sum3/1
  Sum2/1 -> Integrator2/1
  Product/1 -> Sum2/3
  Sum3/1 -> Product/2
  Integrator2/1 -> Product/1, " G(t)"/1
  Sum1/1 -> Integrator1/1

== system final_model/100g.1 ==
  " u(t)" : Inport
  p(t) : Inport  Port=2
  Constant : Constant  Value=p1*Gb
  Constant1 : Constant  Value=p1
  Gain : Gain  Gain=1/V
  Gain1 : Gain  Gain=n
  Gain2 : Gain  Gain=p3
  Gain3 : Gain  Gain=-p2
  Gain4 : Gain  Gain=1/V
  Integrator : Integrator
  Integrator1 : Integrator
  Integrator2 : Integrator  InitialCondition=G0
  Product : Product
  Sum : Sum  Inputs=|+-
  Sum1 : Sum  Inputs=|++
  Sum2 : Sum  Inputs=|++-
  Sum3 : Sum  Inputs=|++
  " G(t)" : Outport
  X(t) : Outport  Port=2
  I(t) : Outport  Port=3
  wires:
  " u(t)"/1 -> Gain/1
  Gain/1 -> Sum/1
  Sum/1 -> Integrator/1
  Integrator/1 -> Gain2/1, I(t)/1, Gain1/1
  Gain1/1 -> Sum/2
  Gain2/1 -> Sum1/1
  Gain3/1 -> Sum1/2
  Integrator1/1 -> Gain3/1, Sum3/2, X(t)/1
  p(t)/1 -> Gain4/1
  Gain4/1 -> Sum2/1
  Constant/1 -> Sum2/2
  Constant1/1 -> Sum3/1
  Sum2/1 -> Integrator2/1
  Product/1 -> Sum2/3
  Sum3/1 -> Product/2
  Integrator2/1 -> Product/1, " G(t)"/1
  Sum1/1 -> Integrator1/1

== system final_model/10g ==
  " u(t)" : Inport
  p(t) : Inport  Port=2
  Constant : Constant  Value=p1*Gb
  Constant1 : Constant  Value=p1
  Gain : Gain  Gain=1/V
  Gain1 : Gain  Gain=n
  Gain2 : Gain  Gain=p3
  Gain3 : Gain  Gain=-p2
  Gain4 : Gain  Gain=1/V
  Integrator : Integrator
  Integrator1 : Integrator
  Integrator2 : Integrator  InitialCondition=G0
  Product : Product
  Sum : Sum  Inputs=|+-
  Sum1 : Sum  Inputs=|++
  Sum2 : Sum  Inputs=|++-
  Sum3 : Sum  Inputs=|++
  " G(t)" : Outport
  X(t) : Outport  Port=2
  I(t) : Outport  Port=3
  wires:
  " u(t)"/1 -> Gain/1
  Gain/1 -> Sum/1
  Sum/1 -> Integrator/1
  Integrator/1 -> Gain2/1, I(t)/1, Gain1/1
  Gain1/1 -> Sum/2
  Gain2/1 -> Sum1/1
  Gain3/1 -> Sum1/2
  Integrator1/1 -> Gain3/1, Sum3/2, X(t)/1
  p(t)/1 -> Gain4/1
  Gain4/1 -> Sum2/1
  Constant/1 -> Sum2/2
  Constant1/1 -> Sum3/1
  Sum2/1 -> Integrator2/1
  Product/1 -> Sum2/3
  Sum3/1 -> Product/2
  Integrator2/1 -> Product/1, " G(t)"/1
  Sum1/1 -> Integrator1/1

== system final_model/10g.1 ==
  " u(t)" : Inport
  p(t) : Inport  Port=2
  Constant : Constant  Value=p1*Gb
  Constant1 : Constant  Value=p1
  Gain : Gain  Gain=1/V
  Gain1 : Gain  Gain=n
  Gain2 : Gain  Gain=p3
  Gain3 : Gain  Gain=-p2
  Gain4 : Gain  Gain=1/V
  Integrator : Integrator
  Integrator1 : Integrator
  Integrator2 : Integrator  InitialCondition=G0
  Product : Product
  Sum : Sum  Inputs=|+-
  Sum1 : Sum  Inputs=|++
  Sum2 : Sum  Inputs=|++-
  Sum3 : Sum  Inputs=|++
  " G(t)" : Outport
  X(t) : Outport  Port=2
  I(t) : Outport  Port=3
  wires:
  " u(t)"/1 -> Gain/1
  Gain/1 -> Sum/1
  Sum/1 -> Integrator/1
  Integrator/1 -> Gain2/1, I(t)/1, Gain1/1
  Gain1/1 -> Sum/2
  Gain2/1 -> Sum1/1
  Gain3/1 -> Sum1/2
  Integrator1/1 -> Gain3/1, Sum3/2, X(t)/1
  p(t)/1 -> Gain4/1
  Gain4/1 -> Sum2/1
  Constant/1 -> Sum2/2
  Constant1/1 -> Sum3/1
  Sum2/1 -> Integrator2/1
  Product/1 -> Sum2/3
  Sum3/1 -> Product/2
  Integrator2/1 -> Product/1, " G(t)"/1
  Sum1/1 -> Integrator1/1

== system final_model/10g1 ==
  " u(t)" : Inport
  p(t) : Inport  Port=2
  Constant : Constant  Value=p1*Gb
  Constant1 : Constant  Value=p1
  Gain : Gain  Gain=1/V
  Gain1 : Gain  Gain=n
  Gain2 : Gain  Gain=p3
  Gain3 : Gain  Gain=-p2
  Gain4 : Gain  Gain=1/V
  Integrator : Integrator
  Integrator1 : Integrator
  Integrator2 : Integrator  InitialCondition=G0
  Product : Product
  Sum : Sum  Inputs=|+-
  Sum1 : Sum  Inputs=|++
  Sum2 : Sum  Inputs=|++-
  Sum3 : Sum  Inputs=|++
  " G(t)" : Outport
  X(t) : Outport  Port=2
  I(t) : Outport  Port=3
  wires:
  " u(t)"/1 -> Gain/1
  Gain/1 -> Sum/1
  Sum/1 -> Integrator/1
  Integrator/1 -> Gain2/1, I(t)/1, Gain1/1
  Gain1/1 -> Sum/2
  Gain2/1 -> Sum1/1
  Gain3/1 -> Sum1/2
  Integrator1/1 -> Gain3/1, Sum3/2, X(t)/1
  p(t)/1 -> Gain4/1
  Gain4/1 -> Sum2/1
  Constant/1 -> Sum2/2
  Constant1/1 -> Sum3/1
  Sum2/1 -> Integrator2/1
  Product/1 -> Sum2/3
  Sum3/1 -> Product/2
  Integrator2/1 -> Product/1, " G(t)"/1
  Sum1/1 -> Integrator1/1

== system final_model/150gg ==
  " u(t)" : Inport
  p(t) : Inport  Port=2
  Constant : Constant  Value=p1*Gb
  Constant1 : Constant  Value=p1
  Gain : Gain  Gain=1/V
  Gain1 : Gain  Gain=n
  Gain2 : Gain  Gain=p3
  Gain3 : Gain  Gain=-p2
  Gain4 : Gain  Gain=1/V
  Integrator : Integrator
  Integrator1 : Integrator
  Integrator2 : Integrator  InitialCondition=G0
  Product : Product
  Sum : Sum  Inputs=|+-
  Sum1 : Sum  Inputs=|++
  Sum2 : Sum  Inputs=|++-
  Sum3 : Sum  Inputs=|++
  " G(t)" : Outport
  X(t) : Outport  Port=2
  I(t) : Outport  Port=3
  wires:
  " u(t)"/1 -> Gain/1
  Gain/1 -> Sum/1
  Sum/1 -> Integrator/1
  Integrator/1 -> Gain2/1, I(t)/1, Gain1/1
  Gain1/1 -> Sum/2
  Gain2/1 -> Sum1/1
  Gain3/1 -> Sum1/2
  Integrator1/1 -> Gain3/1, Sum3/2, X(t)/1
  p(t)/1 -> Gain4/1
  Gain4/1 -> Sum2/1
  Constant/1 -> Sum2/2
  Constant1/1 -> Sum3/1
  Sum2/1 -> Integrator2/1
  Product/1 -> Sum2/3
  Sum3/1 -> Product/2
  Integrator2/1 -> Product/1, " G(t)"/1
  Sum1/1 -> Integrator1/1

== system final_model/200gg ==
  " u(t)" : Inport
  p(t) : Inport  Port=2
  Constant : Constant  Value=p1*Gb
  Constant1 : Constant  Value=p1
  Gain : Gain  Gain=1/V
  Gain1 : Gain  Gain=n
  Gain2 : Gain  Gain=p3
  Gain3 : Gain  Gain=-p2
  Gain4 : Gain  Gain=1/V
  Integrator : Integrator
  Integrator1 : Integrator
  Integrator2 : Integrator  InitialCondition=G0
  Product : Product
  Sum : Sum  Inputs=|+-
  Sum1 : Sum  Inputs=|++
  Sum2 : Sum  Inputs=|++-
  Sum3 : Sum  Inputs=|++
  " G(t)" : Outport
  X(t) : Outport  Port=2
  I(t) : Outport  Port=3
  wires:
  " u(t)"/1 -> Gain/1
  Gain/1 -> Sum/1
  Sum/1 -> Integrator/1
  Integrator/1 -> Gain2/1, I(t)/1, Gain1/1
  Gain1/1 -> Sum/2
  Gain2/1 -> Sum1/1
  Gain3/1 -> Sum1/2
  Integrator1/1 -> Gain3/1, Sum3/2, X(t)/1
  p(t)/1 -> Gain4/1
  Gain4/1 -> Sum2/1
  Constant/1 -> Sum2/2
  Constant1/1 -> Sum3/1
  Sum2/1 -> Integrator2/1
  Product/1 -> Sum2/3
  Sum3/1 -> Product/2
  Integrator2/1 -> Product/1, " G(t)"/1
  Sum1/1 -> Integrator1/1

== system final_model/250gg ==
  " u(t)" : Inport
  p(t) : Inport  Port=2
  Constant : Constant  Value=p1*Gb
  Constant1 : Constant  Value=p1
  Gain : Gain  Gain=1/V
  Gain1 : Gain  Gain=n
  Gain2 : Gain  Gain=p3
  Gain3 : Gain  Gain=-p2
  Gain4 : Gain  Gain=1/V
  Integrator : Integrator
  Integrator1 : Integrator
  Integrator2 : Integrator  InitialCondition=G0
  Product : Product
  Sum : Sum  Inputs=|+-
  Sum1 : Sum  Inputs=|++
  Sum2 : Sum  Inputs=|++-
  Sum3 : Sum  Inputs=|++
  " G(t)" : Outport
  X(t) : Outport  Port=2
  I(t) : Outport  Port=3
  wires:
  " u(t)"/1 -> Gain/1
  Gain/1 -> Sum/1
  Sum/1 -> Integrator/1
  Integrator/1 -> Gain2/1, I(t)/1, Gain1/1
  Gain1/1 -> Sum/2
  Gain2/1 -> Sum1/1
  Gain3/1 -> Sum1/2
  Integrator1/1 -> Gain3/1, Sum3/2, X(t)/1
  p(t)/1 -> Gain4/1
  Gain4/1 -> Sum2/1
  Constant/1 -> Sum2/2
  Constant1/1 -> Sum3/1
  Sum2/1 -> Integrator2/1
  Product/1 -> Sum2/3
  Sum3/1 -> Product/2
  Integrator2/1 -> Product/1, " G(t)"/1
  Sum1/1 -> Integrator1/1

== system final_model/300gg ==
  " u(t)" : Inport
  p(t) : Inport  Port=2
  Constant : Constant  Value=p1*Gb
  Constant1 : Constant  Value=p1
  Gain : Gain  Gain=1/V
  Gain1 : Gain  Gain=n
  Gain2 : Gain  Gain=p3
  Gain3 : Gain  Gain=-p2
  Gain4 : Gain  Gain=1/V
  Integrator : Integrator
  Integrator1 : Integrator
  Integrator2 : Integrator  InitialCondition=G0
  Product : Product
  Sum : Sum  Inputs=|+-
  Sum1 : Sum  Inputs=|++
  Sum2 : Sum  Inputs=|++-
  Sum3 : Sum  Inputs=|++
  " G(t)" : Outport
  X(t) : Outport  Port=2
  I(t) : Outport  Port=3
  wires:
  " u(t)"/1 -> Gain/1
  Gain/1 -> Sum/1
  Sum/1 -> Integrator/1
  Integrator/1 -> Gain2/1, I(t)/1, Gain1/1
  Gain1/1 -> Sum/2
  Gain2/1 -> Sum1/1
  Gain3/1 -> Sum1/2
  Integrator1/1 -> Gain3/1, Sum3/2, X(t)/1
  p(t)/1 -> Gain4/1
  Gain4/1 -> Sum2/1
  Constant/1 -> Sum2/2
  Constant1/1 -> Sum3/1
  Sum2/1 -> Integrator2/1
  Product/1 -> Sum2/3
  Sum3/1 -> Product/2
  Integrator2/1 -> Product/1, " G(t)"/1
  Sum1/1 -> Integrator1/1

== system final_model/40.1g ==
  p(t) : Inport
  u(t) : Inport  Port=2
  Constant : Constant  Value=Gb
  Constant1 : Constant  Value=p1
  Gain : Gain  Gain=1/V
  Gain1 : Gain  Gain=p1
  Gain2 : Gain  Gain=p2
  Gain3 : Gain  Gain=1/V
  Gain4 : Gain  Gain=n
  Gain5 : Gain  Gain=p3
  Integrator : Integrator  InitialCondition=G0
  Integrator1 : Integrator
  Integrator2 : Integrator
  Product : Product
  Product1 : Product
  Sum : Sum  Inputs=|++--
  Sum1 : Sum  Inputs=|+-
  Sum2 : Sum  Inputs=|+-
  G(t) : Outport
  X(t) : Outport  Port=2
  I(t) : Outport  Port=3
  wires:
  Sum2/1 -> Integrator2/1
  Gain3/1 -> Sum2/1
  Sum1/1 -> Integrator1/1
  Integrator2/1 -> Gain4/1, I(t)/1, Gain5/1
  u(t)/1 -> Gain3/1
  Integrator1/1 -> Product1/2, X(t)/1, Gain2/1
  Product/1 -> Sum/2
  Integrator/1 -> G(t)/1, Gain1/1, Product1/1
  Gain5/1 -> Sum1/1
  Sum/1 -> Integrator/1
  Constant1/1 -> Product/2
  Constant/1 -> Product/1
  Gain4/1 -> Sum2/2
  Gain2/1 -> Sum1/2
  Product1/1 -> Sum/3
  Gain1/1 -> Sum/4
  p(t)/1 -> Gain/1
  Gain/1 -> Sum/1

== system final_model/40.1g1 ==
  p(t) : Inport
  u(t) : Inport  Port=2
  Constant : Constant  Value=Gb
  Constant1 : Constant  Value=p1
  Gain : Gain  Gain=1/V
  Gain1 : Gain  Gain=p1
  Gain2 : Gain  Gain=p2
  Gain3 : Gain  Gain=1/V
  Gain4 : Gain  Gain=n
  Gain5 : Gain  Gain=p3
  Integrator : Integrator  InitialCondition=G0
  Integrator1 : Integrator
  Integrator2 : Integrator
  Product : Product
  Product1 : Product
  Sum : Sum  Inputs=|++--
  Sum1 : Sum  Inputs=|+-
  Sum2 : Sum  Inputs=|+-
  G(t) : Outport
  X(t) : Outport  Port=2
  I(t) : Outport  Port=3
  wires:
  Sum2/1 -> Integrator2/1
  Gain3/1 -> Sum2/1
  Sum1/1 -> Integrator1/1
  Integrator2/1 -> Gain4/1, I(t)/1, Gain5/1
  u(t)/1 -> Gain3/1
  Integrator1/1 -> Product1/2, X(t)/1, Gain2/1
  Product/1 -> Sum/2
  Integrator/1 -> G(t)/1, Gain1/1, Product1/1
  Gain5/1 -> Sum1/1
  Sum/1 -> Integrator/1
  Constant1/1 -> Product/2
  Constant/1 -> Product/1
  Gain4/1 -> Sum2/2
  Gain2/1 -> Sum1/2
  Product1/1 -> Sum/3
  Gain1/1 -> Sum/4
  p(t)/1 -> Gain/1
  Gain/1 -> Sum/1
